simulink model "Problem_2"  (R2020b)
settings: Solver=VariableStepAuto  StartTime=0.0  StopTime=10.0  RelTol=1e-3
model workspace (MAT data in the model file):
  B = Simulink.Parameter
  B.Value = 500
  B.DataType = 'auto'
  B.Dimensions = [1 1]
  K1 = Simulink.Parameter
  K1.Value = 300
  K1.DataType = 'auto'
  K1.Dimensions = [1 1]
  K2 = Simulink.Parameter
  K2.Value = 2000
  K2.DataType = 'auto'
  K2.Dimensions = [1 1]
  M1 = Simulink.Parameter
  M1.Value = 1000
  M1.DataType = 'auto'
  M1.Dimensions = [1 1]
  M2 = Simulink.Parameter
  M2.Value = 50
  M2.DataType = 'auto'
  M2.Dimensions = [1 1]
settings Model: Creator=Yeshwanth  LastModifiedBy=Yeshwanth

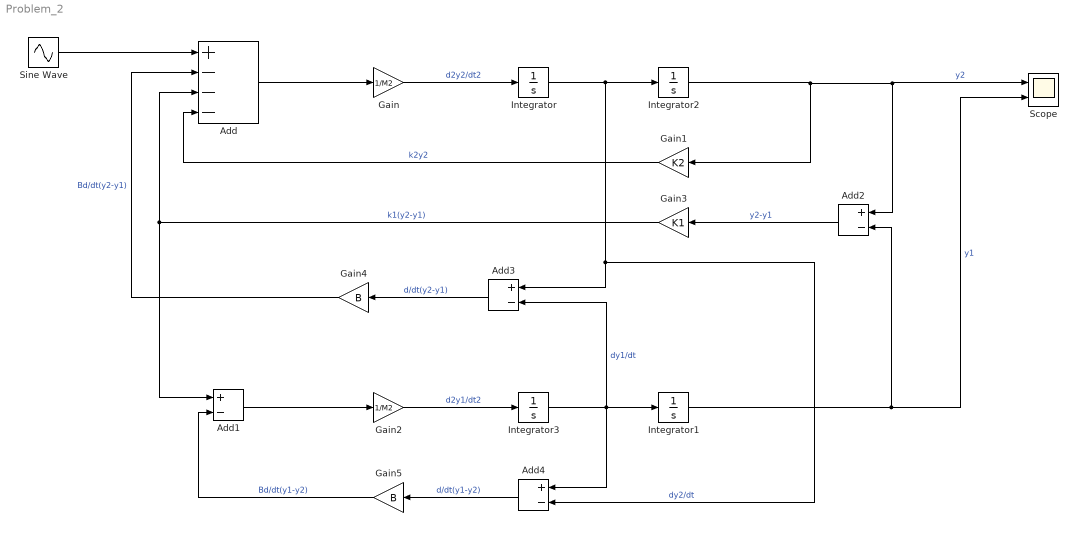
== system Problem_2 ==
  Add : Sum  Inputs=+---
  Add{1..4} (4 alike) : Sum  Inputs=+-
  Gain : Gain  Gain=1/M2
  Gain1 : Gain  Gain=K2
  Gain2 : Gain  Gain=1/M2
  Gain3 : Gain  Gain=K1
  Gain4 : Gain  Gain=B
  Gain5 : Gain  Gain=B
  Integrator{,1..3} (4 alike) : Integrator
  Scope : Scope  NumInputPorts=2
  Sine Wave : Sin  SampleTime=0
  wires:
  Add2/1 -> Gain3/1  "y2-y1"
  Add1/1 -> Gain2/1
  Gain3/1 -> Add1/1, Add/3  "k1(y2-y1)"
  Gain5/1 -> Add1/2  "Bd/dt(y1-y2)"
  Add/1 -> Gain/1
  Gain/1 -> Integrator/1  "d2y2/dt2"
  Integrator2/1 -> Scope/1, Add2/1, Gain1/1  "y2"
  Integrator/1 -> Add4/2, Add3/1, Integrator2/1  "dy2/dt"
  Integrator1/1 -> Add2/2, Scope/2  "y1"
  Gain1/1 -> Add/4  "k2y2"
  Gain4/1 -> Add/2  "Bd/dt(y2-y1)"
  Gain2/1 -> Integrator3/1  "d2y1/dt2"
  Integrator3/1 -> Add4/1, Add3/2, Integrator1/1  "dy1/dt"
  Add3/1 -> Gain4/1  "d/dt(y2-y1)"
  Add4/1 -> Gain5/1  "d/dt(y1-y2)"
  Sine Wave/1 -> Add/1
